simulink model "model_GT"  (R2019b)
settings: Solver=VariableStepAuto  StartTime=0.0  StopTime=nb_time_unit_in_a_simulation/5  RelTol=1e-3
values from neighbouring files (symbols this model uses):
  nb_air_cons = nb_rooms-2    [load_parameters.m]
  nb_boilers = 2    [load_parameters.m]
  nb_radiators = nb_rooms-2    [load_parameters.m]
  nb_second_in_timeunit = 60*5    (= 300)    [full_test.m]
  nb_step_to_fifteen_min = 3    [full_test.m]
  nb_step_to_one_h = 12    [full_test.m]
  nb_step_to_thirty_min = 6    [full_test.m]
  timeunit_in_a_day = 2*6*24    (= 288)    [full_test.m]
undefined symbols (not defined in the file or in its folder): air_mass_kg_rooms, Area_boiler, area_outdoor_rooms, Area_radiators, area_rooms_ground, area_walls_between_rooms, C_air, C_water, Energy_used_by_air_conditioner_for_1_timeunit_in_Watts_vector, Energy_used_by_air_mixer_for_1_timeunit_in_Watts, Energy_used_by_boiler_for_1_timeunit_in_Watts, initial_relative_humidity, initial_temp_water_in_boilers, initial_temperature_rooms, initial_temperature_water_in_radiator, k_boiler_border, k_radiators, k_wall_outdoor_rooms, k_walls_between_rooms, mass_water_radiator, matrix_AC_rooms_locations, matrix_boiler_radiator_connection, matrix_boiler_rooms_locations, matrix_radiator_rooms_locations, nb_humans, nb_rooms, outdoor_max_temp_A, outdoor_max_temp_B, outdoor_min_temp_A, outdoor_min_temp_B, tau_boiler, thickness_boiler, thickness_outdoor_rooms, thickness_radiator_pipes, thickness_walls_between_rooms, Volume_radiators, Volume_rooms, water_weight_in_boiler, watt_generation_of_employe
libraries: dspmtrx3 x15, dspstat3 x6, simulink x2
(part 2 of 2)

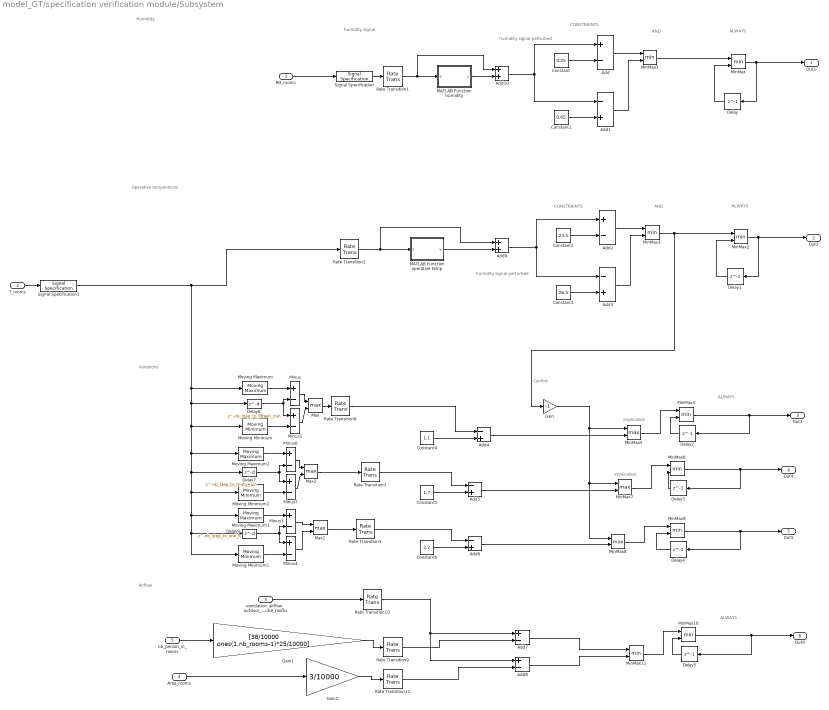
== system model_GT/specification verification module/Subsystem ==
  note: humidity signal perturbed
  note: ALWAYS
  note: implication
  note: AND
  note: implication
  note: humidity signal
  note: Airflow
  note: ALWAYS
  note: AND
  note: Humidity
  note: Operative temperature
  note: Variations
  note: humidity signal perturbed
  note: ALWAYS
  note: Confort
  note: ALWAYS
  note: CONSTRAINTS
  note: CONSTRAINTS
  RH_rooms : Inport  PortDimensions=nb_rooms
  T_rooms : Inport  Port=2  PortDimensions=nb_rooms
  ventilation_airflow_outdoor_air_mcube_rooms : Inport  Port=3  PortDimensions=nb_rooms
  Area_rooms : Inport  Port=4  PortDimensions=nb_rooms
  nb_person_in_rooms : Inport  Port=5  OutDataTypeStr=double  PortDimensions=nb_rooms
  Add{,2,7..8} (4 alike) : Sum  Inputs=+-
  Add{1,3..6} (5 alike) : Sum  Inputs=-+
  Add10 : Sum
  Add9 : Sum
  Constant : Constant  Value=0.25
  Constant1 : Constant  Value=0.65
  Constant2 : Constant  Value=23.5
  Constant3 : Constant  Value=26.5
  Constant4 : Constant  Value=1.1
  Constant5 : Constant  Value=1.7
  Constant6 : Constant  Value=2.2
  Delay{,1..5} (6 alike) : Delay  DelayLength=1  InitialCondition=0
  Delay6 : Delay  DelayLength=nb_step_to_fifteen_min  InitialCondition=27
  Delay7 : Delay  DelayLength=nb_step_to_thirty_min  InitialCondition=27
  Delay8 : Delay  DelayLength=nb_step_to_one_h  InitialCondition=27
  Gain : Gain  Gain=-1
  Gain1 : Gain  Gain=[38/10000 ones(1,nb_rooms-1)*25/10000]
  Gain2 : Gain  Gain=3/10000
  MATLAB Function humidity : MATLAB Function  TreatAsAtomicUnit=on
  MATLAB Function operative temp : MATLAB Function  TreatAsAtomicUnit=on
  Max : MinMax  Function=max  Inputs=2  ZeroCross=off
  Max1 : MinMax  Function=max  Inputs=2  ZeroCross=off
  Max2 : MinMax  Function=max  Inputs=2  ZeroCross=off
  MinMax{,1..4,6,9..11} (9 alike) : MinMax  Inputs=2
  MinMax5 : MinMax  Function=max  Inputs=2
  MinMax7 : MinMax  Function=max  Inputs=2
  MinMax8 : MinMax  Function=max  Inputs=2
  Minus{,1,3..4,6..7} (6 alike) : Sum  Inputs=+-
  Moving Maximum : dspstat3/Moving Maximum  SpecifyWindowLength=on  WindowLength=nb_step_to_fifteen_min  SimulateUsing=Code generation
      settings: SourceProductName=DSP System Toolbox  SourceProductBaseCode=DS
  Moving Maximum1 : dspstat3/Moving Maximum  SpecifyWindowLength=on  WindowLength=nb_step_to_one_h  SimulateUsing=Code generation
      settings: SourceProductName=DSP System Toolbox  SourceProductBaseCode=DS
  Moving Maximum2 : dspstat3/Moving Maximum  SpecifyWindowLength=on  WindowLength=nb_step_to_thirty_min  SimulateUsing=Code generation
      settings: SourceProductName=DSP System Toolbox  SourceProductBaseCode=DS
  Moving Minimum : dspstat3/Moving Minimum  SpecifyWindowLength=on  WindowLength=nb_step_to_fifteen_min  SimulateUsing=Code generation
      settings: SourceProductName=DSP System Toolbox  SourceProductBaseCode=DS
  Moving Minimum1 : dspstat3/Moving Minimum  SpecifyWindowLength=on  WindowLength=nb_step_to_one_h  SimulateUsing=Code generation
      settings: SourceProductName=DSP System Toolbox  SourceProductBaseCode=DS
  Moving Minimum2 : dspstat3/Moving Minimum  SpecifyWindowLength=on  WindowLength=nb_step_to_thirty_min  SimulateUsing=Code generation
      settings: SourceProductName=DSP System Toolbox  SourceProductBaseCode=DS
  Rate Transition{1..3,5,8..11} (8 alike) : RateTransition  OutPortSampleTime=rate
  Signal Specification : SignalSpecification  OutMin=-0.25  OutMax=1.25  Dimensions=nb_rooms
  Signal Specification1 : SignalSpecification  OutMin=-100  OutMax=100  Dimensions=nb_rooms
  Out1 : Outport
  Out2 : Outport  Port=2
  Out3 : Outport  Port=3
  Out4 : Outport  Port=4
  Out5 : Outport  Port=5
  Out6 : Outport  Port=6
  wires:
  Minus1/1 -> Max/2
  Delay5/1 -> MinMax10/2
  Add2/1 -> MinMax3/1
  MinMax10/1 -> Delay5/1, Out6/1
  Delay1/1 -> MinMax2/2
  Minus/1 -> Max/1
  Signal Specification/1 -> Rate Transition1/1
  MinMax7/1 -> MinMax6/1
  T_rooms/1 -> Signal Specification1/1
  Constant1/1 -> Add1/2
  Max1/1 -> Rate Transition5/1
  Constant4/1 -> Add4/2
  Delay4/1 -> MinMax9/2
  Add8/1 -> MinMax11/2
  Rate Transition8/1 -> Add4/1
  MinMax8/1 -> MinMax9/1
  Add3/1 -> MinMax3/2
  MinMax9/1 -> Delay4/1, Out5/1
  Rate Transition11/1 -> Add8/2
  Max2/1 -> Rate Transition3/1
  MinMax1/1 -> MinMax/1
  Rate Transition2/1 -> Add9/1, MATLAB Function operative temp/1(s)
  Gain/1 -> MinMax8/1, MinMax7/1, MinMax5/1
  Minus3/1 -> Max1/1
  Add1/1 -> MinMax1/2
  ventilation_airflow_outdoor_air_mcube_rooms/1 -> Rate Transition10/1
  Rate Transition3/1 -> Add5/1
  Moving Minimum2/1 -> Minus7/2
  Rate Transition5/1 -> Add6/1
  Rate Transition1/1 -> Add10/1, MATLAB Function humidity/1(s)
  MinMax6/1 -> Delay3/1, Out4/1
  MinMax11/1 -> MinMax10/1
  Add9/1 -> Add3/1, Add2/1
  Delay2/1 -> MinMax4/2
  Delay6/1 -> Minus1/1, Minus/2
  MinMax/1 -> Out1/1, Delay/1
  Delay7/1 -> Minus6/2, Minus7/1
  Moving Maximum1/1 -> Minus3/1
  Minus4/1 -> Max1/2
  Signal Specification1/1 -> Moving Maximum/1, Moving Maximum2/1, Delay7/1, Moving Maximum1/1, Delay8/1, Moving Minimum1/1, Moving Minimum2/1, Moving Minimum/1, Delay6/1, Rate Transition2/1
  Moving Maximum2/1 -> Minus6/1
  Max/1 -> Rate Transition8/1
  RH_rooms/1 -> Signal Specification/1
  Constant/1 -> Add/2
  nb_person_in_rooms/1 -> Gain1/1
  Constant3/1 -> Add3/2
  Add6/1 -> MinMax8/2
  Moving Minimum/1 -> Minus1/2
  MinMax5/1 -> MinMax4/1
  Gain1/1 -> Rate Transition9/1
  Constant6/1 -> Add6/2
  Add/1 -> MinMax1/1
  Constant5/1 -> Add5/2
  Delay/1 -> MinMax/2
  Minus7/1 -> Max2/2
  Constant2/1 -> Add2/2
  Gain2/1 -> Rate Transition11/1
  Moving Maximum/1 -> Minus/1
  Delay3/1 -> MinMax6/2
  Area_rooms/1 -> Gain2/1
  Minus6/1 -> Max2/1
  MinMax3/1 -> Gain/1, MinMax2/1
  Delay8/1 -> Minus3/2, Minus4/1
  Moving Minimum1/1 -> Minus4/2
  Add10/1 -> Add1/1, Add/1
  Rate Transition10/1 -> Add8/1, Add7/1
  Add7/1 -> MinMax11/1
  MinMax4/1 -> Delay2/1, Out3/1
  Add5/1 -> MinMax7/2
  MinMax2/1 -> Out2/1, Delay1/1
  Rate Transition9/1 -> Add7/2
  Add4/1 -> MinMax5/2
  MATLAB Function operative temp/1(y) -> Add9/2
  MATLAB Function humidity/1(y) -> Add10/2

== system model_GT/Physical model/Wall heat Exchange module/Value heat exchange outdoor -> rooms ==
  T_rooms : Inport
  outdoor : Inport  Port=2
  Gain : Gain  Gain=area_outdoor_rooms
  Gain1 : Gain  Gain=k_wall_outdoor_rooms
  Gain2 : Gain  Gain=ones(nb_rooms,1)./thickness_outdoor_rooms
  Sum : Sum  Inputs=|+-
  Q_outdoor_to_rooms : Outport
  wires:
  T_rooms/1 -> Sum/2
  outdoor/1 -> Sum/1
  Sum/1 -> Gain/1
  Gain/1 -> Gain1/1
  Gain1/1 -> Gain2/1
  Gain2/1 -> Q_outdoor_to_rooms/1

== system model_GT/Physical model/Wall heat Exchange module/Value heat exchange within building ==
  "T_rooms " : Inport
  Constant : Constant  Value=diag(ones(nb_rooms,1))
  Gain3 : Gain  Gain=area_walls_between_rooms
  Gain4 : Gain  Gain=k_walls_between_rooms
  Gain8 : Gain  Gain=ones(nb_rooms,nb_rooms)./thickness_walls_between_rooms
  MATRIX WITH ROOM TEMPERATURE DIFFERENCE The area matrix after handles the case of non-adjacent rooms : dspmtrx3/Array-Vector Multiply  mode=Mute  saveAsFlag=0  Dimension=2  V_Source=Input port  V_VectFromMask=[0.5 0.25]  roundingMode=Floor  overflowMode=off  firstCoeffSignedness=Auto  firstCoeffDataTypeStr=Inherit: Same word length as input  firstCoeffMin=[]  firstCoeffMax=[]  firstCoeffLastDataTypeStr=Inherit: Same word length as input  prodOutputSignedness=Auto  accumSignedness=Auto  outputSignedness=Auto  outputDataTypeStr=Inherit: Same as product output  outputMin=[]  outputMax=[]  outputLastDataTypeStr=Inherit: Same as product output
      settings: SourceProductName=DSP System Toolbox  SourceProductBaseCode=DS
  Sum of Elements : Sum  Inputs=+  CollapseMode=Specified dimension  CollapseDim=2
  Q_in_building_to_rooms : Outport
  wires:
  Gain4/1 -> Gain8/1
  Gain3/1 -> Gain4/1
  MATRIX WITH ROOM TEMPERATURE DIFFERENCE The area matrix after handles the case of non-adjacent rooms/1 -> Gain3/1
  Gain8/1 -> Sum of Elements/1
  Sum of Elements/1 -> Q_in_building_to_rooms/1
  Constant/1 -> MATRIX WITH ROOM TEMPERATURE DIFFERENCE The area matrix after handles the case of non-adjacent rooms/1
  "T_rooms "/1 -> MATRIX WITH ROOM TEMPERATURE DIFFERENCE The area matrix after handles the case of non-adjacent rooms/2

== matlab function model_GT/specification verification module/Subsystem/MATLAB Function operative temp ==
  data: s input; y output
function y = fcn(s)
	
    y = zeros(size(s,1),1);

    function yy = fbis(ee)
        left = ee-23.5; 
        right = 26.5-ee;    
        yy = min(left,right); % AND
    end

    for i=1:size(s,1)
        ss = s(i);
        [a b] =  fminbnd(@fbis,ss-1,ss+1);  
        y(i)=a-ss;
    end
    
end

== matlab function model_GT/specification verification module/Subsystem/MATLAB Function humidity ==
  data: s input; y output
function y = fcn(s)
    
    y = zeros(size(s,1),1);
    
    function yy = fbis(ee)
        left = ee-0.25; 
        right = 0.65-ee;    
        yy = min(left,right); % AND
    end

    
    for i=1:size(s,1)
        ss = s(i);
        [a b] =  fminbnd(@fbis,ss-0.1,ss+0.1);  
        y(i)=a-ss;
    end
    
end
